simulink model "real_controller_A_2015B"  (R2015b)
settings: Solver=VariableStepAuto  StartTime=0.0  StopTime=sim_run  RelTol=1e-3
undefined symbols (not defined in the file): sigbuilder_block, Standard_Devices, UDP_Protocol, zh_step
libraries: simulink x4, sldrtlib x2
settings Model: Creator=Anony  LastModifiedBy=Anony

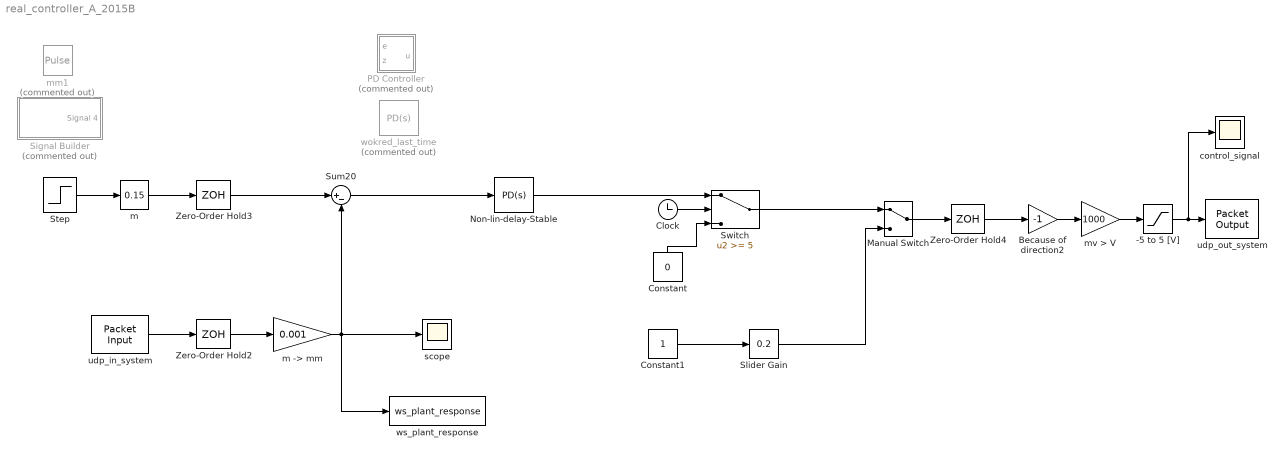
== system real_controller_A_2015B ==
  -5 to 5 [V] : Saturate  UpperLimit=5  LowerLimit=-5
  Because of direction2 : Gain  Gain=-1
  Clock : Clock
  Constant : Constant  Value=0
  Constant1 : Constant
  Manual Switch : ManualSwitch
  Non-lin-delay-Stable : simulink/Continuous/PID Controller  Controller=PD  TimeDomain=Continuous-time  SampleTime=-1  IntegratorMethod=Forward Euler  FilterMethod=Forward Euler  Form=Parallel  UseFilter=on  ControllerParametersSource=internal  P=0.008  I=0.0175856984919557  D=0.0001  N=100  InitialConditionSource=internal  InitialConditionForIntegrator=0  InitialConditionForFilter=0  ExternalReset=none  LimitOutput=off  UpperSaturationLimit=5/1000  LowerSaturationLimit=-5/1000  LinearizeAsGain=on  AntiWindupMode=none  Kb=1  TrackingMode=off  Kt=1  PParamMin=[]  PParamMax=[]  IParamMin=[]  IParamMax=[]  DParamMin=[]  DParamMax=[]  NParamMin=[]  NParamMax=[]  KbParamMin=[]  KbParamMax=[]  KtParamMin=[]  KtParamMax=[]  POutMin=[]  POutMax=[]  IOutMin=[]  IOutMax=[]  DOutMin=[]  DOutMax=[]  NOutMin=[]  NOutMax=[]  KbOutMin=[]  KbOutMax=[]  KtOutMin=[]  KtOutMax=[]  IntegratorOutMin=[]  IntegratorOutMax=[]  FilterOutMin=[]  FilterOutMax=[]  SumOutMin=[]  SumOutMax=[]  SumI1OutMin=[]  SumI1OutMax=[]  SumI2OutMin=[]  SumI2OutMax=[]  SumI3OutMin=[]  SumI3OutMax=[]  SumDOutMin=[]  SumDOutMax=[]  SaturationOutMin=[]  SaturationOutMax=[]  IntegratorContinuousStateAttributes=''  IntegratorStateMustResolveToSignalObject=off  IntegratorRTWStateStorageClass=Auto  FilterContinuousStateAttributes=''  FilterStateMustResolveToSignalObject=off  FilterRTWStateStorageClass=Auto  DifferentiatorICPrevScaledInput=0  DifferentiatorOutMin=[]  DifferentiatorOutMax=[]
  PD Controller : Subsystem  Commented=on
  Signal Builder : Subsystem  Tag=STV Subsys  Commented=on  LoadFcn=sigbuilder_block('load');  StartFcn=sigbuilder_block('start');  StopFcn=sigbuilder_block('stop');  ClipboardFcn=sigbuilder_block('clipboard');  mask(Sigbuilder block){}
      mask help: Simulink:masks:SigbuilderBlock_MD
      mask init:
      | if ~strcmp(get_param(bdroot(gcbh),'SimulationStatus'),'stopped') tuvar = sigbuilder_block('maskInit'); end
      settings: CopyFcn=sigbuilder_block('copy');  DeleteFcn=sigbuilder_block('delete');  ModelCloseFcn=sigbuilder_block('modelClose');  PreSaveFcn=sigbuilder_block('preSave');  PauseFcn=sigbuilder_block('pause');  ContinueFcn=sigbuilder_block('continue');  NameChangeFcn=sigbuilder_block('namechange');  OpenFcn=sigbuilder_block('open',[267 41.1429 550.714 363 ]);  CloseFcn=sigbuilder_block('close');
      mask Display: plot(0, 0, 100, 100,[2, 2, 32, 32, 2], [68, 8, 8, 68, 68],[32, 2], [38, 38], [32, 19, 2],[53, 60, 44], [32, 17, 17, 2],[16, 16, 31, 31]);txt = getActiveGroup(gcbh);text(2, 100, txt,'verticalAlignment', 'top');
  Slider Gain : simulink/Math Operations/Slider Gain  low=0  gain=0.2  high=0.3
  Step : Step  Time=5  SampleTime=0
  Sum20 : Sum  Inputs=|+-
  Switch : Switch  Threshold=5
  Zero-Order Hold2 : ZeroOrderHold  SampleTime=zh_step
  Zero-Order Hold3 : ZeroOrderHold  SampleTime=zh_step
  Zero-Order Hold4 : ZeroOrderHold  SampleTime=zh_step
  control_signal : Scope
  m : simulink/Math Operations/Slider Gain  low=0  gain=0.15  high=0.6
  "m -> mm" : Gain  Gain=0.001
  mm1 : DiscretePulseGenerator  Commented=on  PulseType=Time based  Amplitude=150  Period=20  PulseWidth=50
  mv > V : Gain  Gain=1000
  scope : Scope
  udp_in_system : sldrtlib/Packet Input  SampleTime=0.001  MaxMissedTicks=inf  ShowMissedTicks=off  YieldWhenWaiting=off  DrvName=Standard_Devices/UDP_Protocol  DrvAddress=28500  DrvOptions=[2468389192 28500]  PacketSize=8  DataTypes='double'  ShowReady=off  ShowError=off  PacketID=1  ByteOrder=1  ShowTimestamp=off
  udp_out_system : sldrtlib/Packet Output  SampleTime=0.01  MaxMissedTicks=inf  ShowMissedTicks=off  YieldWhenWaiting=off  DrvName=Standard_Devices/UDP_Protocol  DrvAddress=27500  DrvOptions=[2468389192 27500]  PacketSize=8  DataTypes='double'  ShowReady=off  ShowError=off  PacketID=1  ByteOrder=1  InitialValue=[]  FinalValue=[]
      settings: AttributesFormatString=Standard Devices\nUDP Protocol [6B6Ch]
  wokred_last_time : simulink/Continuous/PID Controller  Commented=on  Controller=PD  TimeDomain=Continuous-time  SampleTime=-1  IntegratorMethod=Forward Euler  FilterMethod=Forward Euler  Form=Parallel  UseFilter=on  ControllerParametersSource=internal  P=0.0142  I=0.0175856984919557  D=0.0001  N=100  InitialConditionSource=internal  InitialConditionForIntegrator=0  InitialConditionForFilter=0  ExternalReset=none  LimitOutput=on  UpperSaturationLimit=5/1000  LowerSaturationLimit=-5/1000  LinearizeAsGain=on  AntiWindupMode=none  Kb=1  TrackingMode=off  Kt=1  PParamMin=[]  PParamMax=[]  IParamMin=[]  IParamMax=[]  DParamMin=[]  DParamMax=[]  NParamMin=[]  NParamMax=[]  KbParamMin=[]  KbParamMax=[]  KtParamMin=[]  KtParamMax=[]  POutMin=[]  POutMax=[]  IOutMin=[]  IOutMax=[]  DOutMin=[]  DOutMax=[]  NOutMin=[]  NOutMax=[]  KbOutMin=[]  KbOutMax=[]  KtOutMin=[]  KtOutMax=[]  IntegratorOutMin=[]  IntegratorOutMax=[]  FilterOutMin=[]  FilterOutMax=[]  SumOutMin=[]  SumOutMax=[]  SumI1OutMin=[]  SumI1OutMax=[]  SumI2OutMin=[]  SumI2OutMax=[]  SumI3OutMin=[]  SumI3OutMax=[]  SumDOutMin=[]  SumDOutMax=[]  SaturationOutMin=[]  SaturationOutMax=[]  IntegratorContinuousStateAttributes=''  IntegratorStateMustResolveToSignalObject=off  IntegratorRTWStateStorageClass=Auto  FilterContinuousStateAttributes=''  FilterStateMustResolveToSignalObject=off  FilterRTWStateStorageClass=Auto  DifferentiatorICPrevScaledInput=0  DifferentiatorOutMin=[]  DifferentiatorOutMax=[]
  ws_plant_response : ToWorkspace  VariableName=ws_plant_response  SaveFormat=Timeseries  SampleTime=-1
  wires:
  Step/1 -> m/1
  Sum20/1 -> Non-lin-delay-Stable/1
  udp_in_system/1 -> Zero-Order Hold2/1
  m/1 -> Zero-Order Hold3/1
  Non-lin-delay-Stable/1 -> Switch/1
  Zero-Order Hold2/1 -> "m -> mm"/1
  Zero-Order Hold3/1 -> Sum20/1
  "m -> mm"/1 -> Sum20/2, ws_plant_response/1, scope/1
  Constant/1 -> Switch/3
  Clock/1 -> Switch/2
  Switch/1 -> Manual Switch/1
  Constant1/1 -> Slider Gain/1
  Slider Gain/1 -> Manual Switch/2
  Zero-Order Hold4/1 -> Because of direction2/1
  Manual Switch/1 -> Zero-Order Hold4/1
  Because of direction2/1 -> mv > V/1
  mv > V/1 -> -5 to 5 [V]/1
  -5 to 5 [V]/1 -> control_signal/1, udp_out_system/1

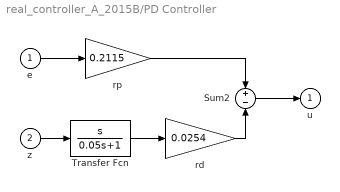
== system real_controller_A_2015B/PD Controller ==
  e : Inport
  z : Inport  Port=2
  Sum2 : Sum  Inputs=+|-
  Transfer Fcn : TransferFcn  Numerator=[1 0]  Denominator=[0.05 1]
  rd : Gain  Gain=0.0254
  rp : Gain  Gain=0.2115
  u : Outport
  wires:
  rp/1 -> Sum2/1
  z/1 -> Transfer Fcn/1
  e/1 -> rp/1
  Transfer Fcn/1 -> rd/1
  rd/1 -> Sum2/2
  Sum2/1 -> u/1

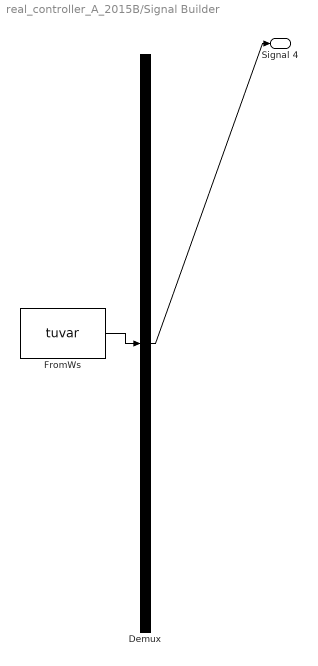
== system real_controller_A_2015B/Signal Builder ==
  Demux : Demux  Tag=STV Demux  Outputs=1
  FromWs : FromWorkspace  Tag=STV FromWs  VariableName=tuvar  SampleTime=0
      SigBuilderData=|
      | common.afterFinalStr = 'Extrapolate'
      | common.sampleTime = 0
      | dataSet.timeRange = [0 60]
      | dataSet.name = 'Group 1'
      | sbobj.Groups.Name = 'Group 1'
      | sbobj.Groups.Signals.Name = 'Signal 4'
      | sbobj.Groups.Signals.XData = [0 20 20 30 30 40 40 50 50 60]
      | sbobj.Groups.Signals.YData = [0 2 500 500 0 0 500 502 0 2]
      | sbobj.Groups.TimeRange = [0 60]
  Signal 4 : Outport  Tag=STV Outport
  wires:
  FromWs/1 -> Demux/1
  Demux/1 -> Signal 4/1
